simulink model "SolutionP2"  (Simulink 9.2)
settings: Solver=VariableStepAuto  StartTime=0.0  StopTime=tmax  MaxStep=0.1  RelTol=1e-3
values from neighbouring files (symbols this model uses):
  A = sys.A    [SolutionP1.m]    (also in SolutionP22.m = [0, -a0;1, -a1]; SolutionP2KalmanFilter.m = [0 -a2; SolutionP31.m = [0, -a0;1, -a1])
  a0 = 1    [SolutionP1.m]    (also in SolutionP22.m; SolutionP31.m)
  a1 = 0.5    [SolutionP1.m]    (also in SolutionP22.m = 0.2; SolutionP2KalmanFilter.m = -1.5; SolutionP31.m = 0.2)
  B = [b0; 0]    [SolutionP22.m]    (also in SolutionP2KalmanFilter.m = [0 b0]'; SolutionP31.m)
  b0 = 1    [SolutionP1.m]    (also in SolutionP22.m; SolutionP2KalmanFilter.m = 0.9; SolutionP31.m)
  C = [0 1]    [SolutionP22.m]    (also in SolutionP2KalmanFilter.m = [0 1]'; SolutionP31.m)
  L = [.2; .1]    [SolutionP22.m]    (also in SolutionP2KalmanFilter.m = 2; SolutionP31.m)
settings Model: Creator=raphael  LastModifiedBy=raphael
settings DataIOCC: LimitDataPoints=off  SaveFormat=Dataset  SignalLoggingSaveFormat=Dataset
settings OptimizationCC: LifeSpan=auto
settings DebuggingCC: UnderspecifiedInitializationDetection=Simplified  MergeDetectMultiDrivingBlocksExec=error  FcnCallInpInsideContextMsg=error  StateNameClashWarn=none  SFUnexpectedBacktrackingDiag=error  SFNoUnconditionalDefaultTransitionDiag=error  SFExecutionAtInitializationDiag=warning
settings HardwareCC: ProdBitPerPointer=64  ProdBitPerSizeT=64  ProdBitPerPtrDiffT=64  ProdLargestAtomicFloat=Float  ProdIntDivRoundTo=Zero  ProdEndianess=LittleEndian  ProdWordSize=64  ProdHWDeviceType=Intel->x86-64 (Windows64)
settings ModelReferenceCC: PropagateSignalLabelsOutOfModel=on
settings SFSimCC: SimUseLocalCustomCode=on
settings RTWCC: RTWUseLocalCustomCode=on
settings CodeAppCC: StateflowObjectComments=off
settings GRTTargetCC: TargetLangStandard=C99 (ISO)  GeneratePreprocessorConditionals=Use local settings  CombineOutputUpdateFcns=on  GRTInterface=off
settings ConfigComp: CovMetricSettings=dwe  CovHtmlReporting=off  CovSaveCumulativeToWorkspaceVar=off  CovSaveSingleToWorkspaceVar=off  CovExternalEMLEnable=on

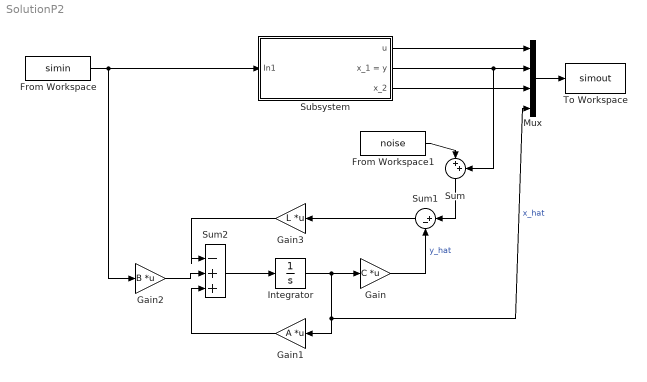
== system SolutionP2 ==
  From Workspace : FromWorkspace  VariableName=simin  SampleTime=0
  From Workspace1 : FromWorkspace  VariableName=noise  SampleTime=0
  Gain : Gain  Gain=C  Multiplication=Matrix(K*u) (u vector)
  Gain1 : Gain  Gain=A  Multiplication=Matrix(K*u) (u vector)
  Gain2 : Gain  Gain=B  Multiplication=Matrix(K*u) (u vector)
  Gain3 : Gain  Gain=L  Multiplication=Matrix(K*u)
  Integrator : Integrator
  Mux : Mux
  Subsystem : Subsystem
  Sum : Sum  Inputs=|++
  Sum1 : Sum  Inputs=|+-
  Sum2 : Sum  Inputs=|-++
  To Workspace : ToWorkspace  VariableName=simout  SaveFormat=Timeseries  SampleTime=-1
  wires:
  Mux/1 -> To Workspace/1
  From Workspace/1 -> Gain2/1, Subsystem/1(In1)
  Subsystem/1(u) -> Mux/1
  Subsystem/2(x_1 = y) -> Sum/2, Mux/2
  Subsystem/3(x_2) -> Mux/3
  From Workspace1/1 -> Sum/1
  Sum/1 -> Sum1/1
  Gain/1 -> Sum1/2  "y_hat"
  Integrator/1 -> Gain1/1, Mux/4, Gain/1  "x_hat"
  Sum2/1 -> Integrator/1
  Gain1/1 -> Sum2/3
  Gain2/1 -> Sum2/2
  Sum1/1 -> Gain3/1
  Gain3/1 -> Sum2/1

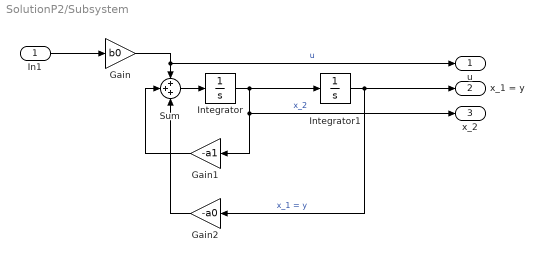
== system SolutionP2/Subsystem ==
  In1 : Inport
  Gain : Gain  Gain=b0
  Gain1 : Gain  Gain=-a1
  Gain2 : Gain  Gain=-a0
  Integrator : Integrator
  Integrator1 : Integrator
  Sum : Sum  Inputs=+++
  u : Outport
  x_1 = y : Outport  Port=2
  x_2 : Outport  Port=3
  wires:
  Gain2/1 -> Sum/3
  Sum/1 -> Integrator/1
  Integrator/1 -> Integrator1/1, Gain1/1, x_2/1  "x_2"
  In1/1 -> Gain/1
  Integrator1/1 -> x_1 = y/1, Gain2/1  "x_1 = y"
  Gain1/1 -> Sum/2
  Gain/1 -> u/1, Sum/1  "u"
